simulink model "MODL1x"  (Simulink 5.0)
settings: Solver=ode45  StartTime=0.0  StopTime=2.0  RelTol=1e-3
settings Model: LastModifiedBy=User  BlockReductionOpt=off  BooleanDataType=off

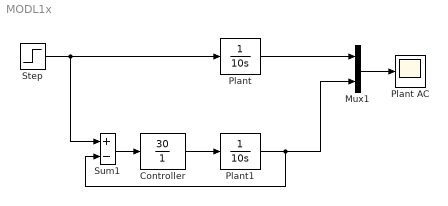
== system MODL1x ==
  Controller : TransferFcn  Numerator=[30]  Denominator=[0 1]
  Mux1 : Mux  Inputs=2
  Plant : TransferFcn  Denominator=[10 0]
  Plant AC : Scope
      settings: YMin=-5e+283  YMax=9e+284
  Plant1 : TransferFcn  Denominator=[10 0]
  Step : Step  Time=0.1  SampleTime=0
  Sum1 : Sum  Inputs=+-  SaturateOnIntegerOverflow=on  InputSameDT=on
  wires:
  Step/1 -> Sum1/1, Plant/1
  Plant/1 -> Mux1/1
  Sum1/1 -> Controller/1
  Controller/1 -> Plant1/1
  Plant1/1 -> Sum1/2, Mux1/2
  Mux1/1 -> Plant AC/1
